simulink model "Neur_PID_sys"  (R2021a)
settings: Solver=FixedStepAuto  StartTime=0.0  StopTime=300  FixedStep=0.01  RelTol=1e-3
settings Model: Creator=WU  LastModifiedBy=WU

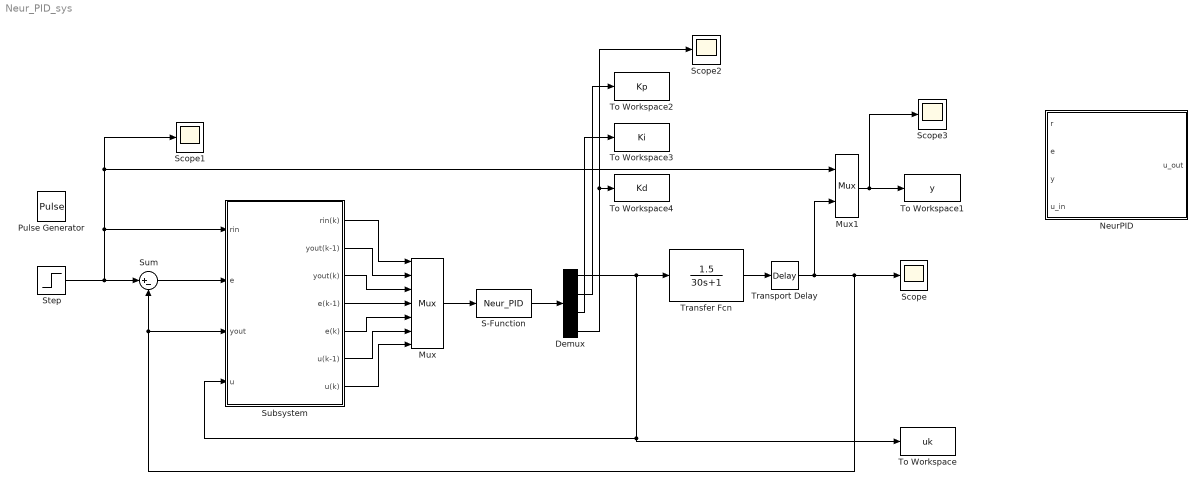
== system Neur_PID_sys ==
  Demux : Demux
  Mux : Mux  Inputs=7
  Mux1 : Mux  Inputs=2
  NeurPID : Subsystem
  Pulse Generator : DiscretePulseGenerator  PulseType=Time based  Period=10  PulseWidth=5
  S-Function : S-Function  FunctionName=Neur_PID  SFunctionDeploymentMode=off  EnableBusSupport=off
  Scope{,1..3} (4 alike) : Scope
  Step : Step  SampleTime=0  ZeroCross=off
  Subsystem : Subsystem
  Sum : Sum  Inputs=|+-
  To Workspace : ToWorkspace  VariableName=uk  SaveFormat=Structure With Time  SampleTime=-1
  To Workspace1 : ToWorkspace  VariableName=y  SaveFormat=Structure With Time  SampleTime=-1
  To Workspace2 : ToWorkspace  VariableName=Kp  SaveFormat=Structure With Time  SampleTime=-1
  To Workspace3 : ToWorkspace  VariableName=Ki  SaveFormat=Structure With Time  SampleTime=-1
  To Workspace4 : ToWorkspace  VariableName=Kd  SaveFormat=Structure With Time  SampleTime=-1
  Transfer Fcn : TransferFcn  Numerator=[1.5]  Denominator=[30 1]
  Transport Delay : TransportDelay  DelayTime=10  BufferSize=100000
  wires:
  Demux/2 -> To Workspace2/1
  Subsystem/6(u(k-1)) -> Mux/6
  Demux/3 -> To Workspace3/1
  Step/1 -> Scope1/1, Mux1/1, Subsystem/1(rin), Sum/1
  Transfer Fcn/1 -> Transport Delay/1
  Mux1/1 -> Scope3/1, To Workspace1/1
  Sum/1 -> Subsystem/2(e)
  Transport Delay/1 -> Mux1/2, Scope/1, Subsystem/3(yout), Sum/2
  Subsystem/1(rin(k)) -> Mux/1
  Subsystem/3(yout(k)) -> Mux/3
  Subsystem/5(e(k)) -> Mux/5
  Subsystem/4(e(k-1)) -> Mux/4
  Demux/1 -> Subsystem/4(u), To Workspace/1, Transfer Fcn/1
  S-Function/1 -> Demux/1
  Demux/4 -> Scope2/1, To Workspace4/1
  Subsystem/2(yout(k-1)) -> Mux/2
  Mux/1 -> S-Function/1
  Subsystem/7(u(k)) -> Mux/7

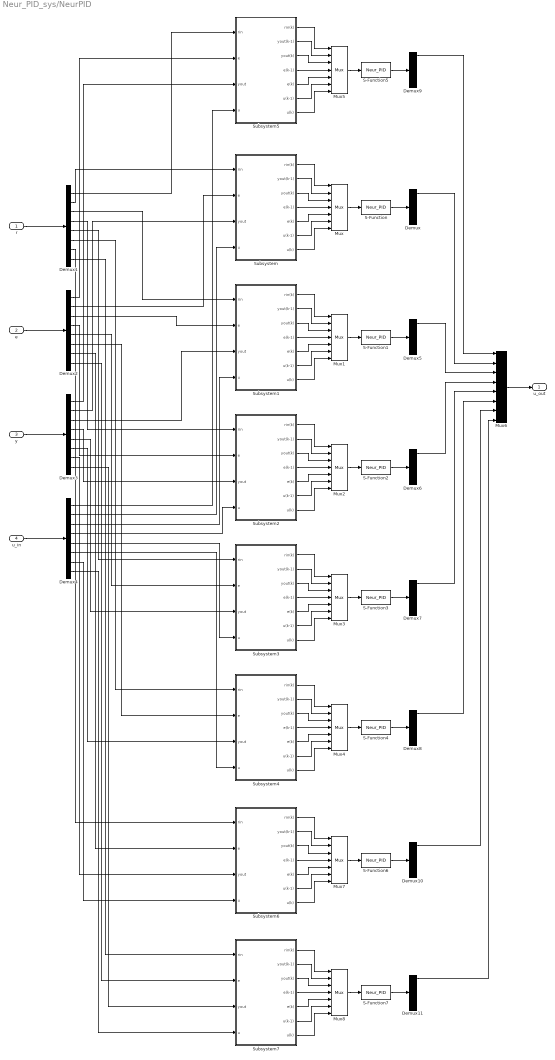
== system Neur_PID_sys/NeurPID ==
  r : Inport
  e : Inport  Port=2
  y : Inport  Port=3
  u_in : Inport  Port=4
  Demux{,5..11} (8 alike) : Demux
      settings: DisplayOption=none
  Demux{1..4} (4 alike) : Demux  Outputs=8
      settings: DisplayOption=none
  Mux{,1..5,7..8} (8 alike) : Mux  Inputs=7
  Mux6 : Mux  Inputs=8
  S-Function{,1..7} (8 alike) : S-Function  FunctionName=Neur_PID  SFunctionDeploymentMode=off  EnableBusSupport=off
  Subsystem : Subsystem
  Subsystem1 : Subsystem
  Subsystem2 : Subsystem
  Subsystem3 : Subsystem
  Subsystem4 : Subsystem
  Subsystem5 : Subsystem
  Subsystem6 : Subsystem
  Subsystem7 : Subsystem
  u_out : Outport
  wires:
  Mux/1 -> S-Function/1
  Subsystem/5(e(k)) -> Mux/5
  S-Function/1 -> Demux/1
  Subsystem/7(u(k)) -> Mux/7
  Subsystem/3(yout(k)) -> Mux/3
  Subsystem/1(rin(k)) -> Mux/1
  Subsystem/6(u(k-1)) -> Mux/6
  Subsystem/4(e(k-1)) -> Mux/4
  Subsystem/2(yout(k-1)) -> Mux/2
  r/1 -> Demux1/1
  e/1 -> Demux2/1
  y/1 -> Demux3/1
  u_in/1 -> Demux4/1
  Subsystem1/4(e(k-1)) -> Mux1/4
  Subsystem1/6(u(k-1)) -> Mux1/6
  Subsystem1/3(yout(k)) -> Mux1/3
  S-Function1/1 -> Demux5/1
  Mux1/1 -> S-Function1/1
  Subsystem1/1(rin(k)) -> Mux1/1
  Subsystem1/7(u(k)) -> Mux1/7
  Subsystem1/5(e(k)) -> Mux1/5
  Subsystem1/2(yout(k-1)) -> Mux1/2
  Subsystem2/4(e(k-1)) -> Mux2/4
  Subsystem2/6(u(k-1)) -> Mux2/6
  Subsystem2/3(yout(k)) -> Mux2/3
  S-Function2/1 -> Demux6/1
  Mux2/1 -> S-Function2/1
  Subsystem2/1(rin(k)) -> Mux2/1
  Subsystem2/7(u(k)) -> Mux2/7
  Subsystem2/5(e(k)) -> Mux2/5
  Subsystem2/2(yout(k-1)) -> Mux2/2
  Subsystem3/4(e(k-1)) -> Mux3/4
  Subsystem3/6(u(k-1)) -> Mux3/6
  Subsystem3/3(yout(k)) -> Mux3/3
  S-Function3/1 -> Demux7/1
  Mux3/1 -> S-Function3/1
  Subsystem3/1(rin(k)) -> Mux3/1
  Subsystem3/7(u(k)) -> Mux3/7
  Subsystem3/5(e(k)) -> Mux3/5
  Subsystem3/2(yout(k-1)) -> Mux3/2
  Subsystem4/4(e(k-1)) -> Mux4/4
  Subsystem4/6(u(k-1)) -> Mux4/6
  Subsystem4/3(yout(k)) -> Mux4/3
  S-Function4/1 -> Demux8/1
  Mux4/1 -> S-Function4/1
  Subsystem4/1(rin(k)) -> Mux4/1
  Subsystem4/7(u(k)) -> Mux4/7
  Subsystem4/5(e(k)) -> Mux4/5
  Subsystem4/2(yout(k-1)) -> Mux4/2
  Subsystem5/4(e(k-1)) -> Mux5/4
  Subsystem5/6(u(k-1)) -> Mux5/6
  Subsystem5/3(yout(k)) -> Mux5/3
  S-Function5/1 -> Demux9/1
  Mux5/1 -> S-Function5/1
  Subsystem5/1(rin(k)) -> Mux5/1
  Subsystem5/7(u(k)) -> Mux5/7
  Subsystem5/5(e(k)) -> Mux5/5
  Subsystem5/2(yout(k-1)) -> Mux5/2
  Demux1/1 -> Subsystem5/1(rin)
  Demux1/2 -> Subsystem/1(rin)
  Demux1/3 -> Subsystem1/1(rin)
  Demux1/4 -> Subsystem2/1(rin)
  Demux1/5 -> Subsystem3/1(rin)
  Demux1/6 -> Subsystem4/1(rin)
  Demux2/1 -> Subsystem5/2(e)
  Demux2/2 -> Subsystem/2(e)
  Demux2/3 -> Subsystem1/2(e)
  Demux2/4 -> Subsystem2/2(e)
  Demux2/5 -> Subsystem3/2(e)
  Demux2/6 -> Subsystem4/2(e)
  Demux3/1 -> Subsystem5/3(yout)
  Demux3/2 -> Subsystem/3(yout)
  Demux3/3 -> Subsystem1/3(yout)
  Demux3/4 -> Subsystem2/3(yout)
  Demux3/5 -> Subsystem3/3(yout)
  Demux3/6 -> Subsystem4/3(yout)
  Demux4/1 -> Subsystem5/4(u)
  Demux4/2 -> Subsystem/4(u)
  Demux4/3 -> Subsystem1/4(u)
  Demux4/4 -> Subsystem2/4(u)
  Demux4/5 -> Subsystem3/4(u)
  Demux4/6 -> Subsystem4/4(u)
  Mux6/1 -> u_out/1
  Demux9/1 -> Mux6/1
  Demux/1 -> Mux6/2
  Demux5/1 -> Mux6/3
  Demux6/1 -> Mux6/4
  Demux7/1 -> Mux6/5
  Demux8/1 -> Mux6/6
  Mux7/1 -> S-Function6/1
  Subsystem6/5(e(k)) -> Mux7/5
  Subsystem6/6(u(k-1)) -> Mux7/6
  Subsystem6/2(yout(k-1)) -> Mux7/2
  Subsystem6/3(yout(k)) -> Mux7/3
  Subsystem6/7(u(k)) -> Mux7/7
  Subsystem6/4(e(k-1)) -> Mux7/4
  S-Function6/1 -> Demux10/1
  Subsystem6/1(rin(k)) -> Mux7/1
  Mux8/1 -> S-Function7/1
  Subsystem7/5(e(k)) -> Mux8/5
  Subsystem7/6(u(k-1)) -> Mux8/6
  Subsystem7/2(yout(k-1)) -> Mux8/2
  Subsystem7/3(yout(k)) -> Mux8/3
  Subsystem7/7(u(k)) -> Mux8/7
  Subsystem7/4(e(k-1)) -> Mux8/4
  S-Function7/1 -> Demux11/1
  Subsystem7/1(rin(k)) -> Mux8/1
  Demux1/7 -> Subsystem6/1(rin)
  Demux2/7 -> Subsystem6/2(e)
  Demux3/7 -> Subsystem6/3(yout)
  Demux4/7 -> Subsystem6/4(u)
  Demux1/8 -> Subsystem7/1(rin)
  Demux2/8 -> Subsystem7/2(e)
  Demux3/8 -> Subsystem7/3(yout)
  Demux4/8 -> Subsystem7/4(u)
  Demux10/1 -> Mux6/7
  Demux11/1 -> Mux6/8

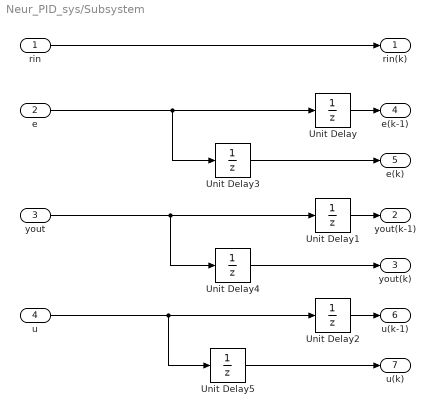
== system Neur_PID_sys/Subsystem ==
  rin : Inport
  e : Inport  Port=2
  yout : Inport  Port=3
  u : Inport  Port=4
  Unit Delay{,1..5} (6 alike) : UnitDelay  SampleTime=-1  HasFrameUpgradeWarning=on
  rin(k) : Outport
  yout(k-1) : Outport  Port=2
  yout(k) : Outport  Port=3
  e(k-1) : Outport  Port=4
  e(k) : Outport  Port=5
  u(k-1) : Outport  Port=6
  u(k) : Outport  Port=7
  wires:
  rin/1 -> rin(k)/1
  Unit Delay/1 -> e(k-1)/1
  Unit Delay1/1 -> yout(k-1)/1
  Unit Delay2/1 -> u(k-1)/1
  Unit Delay3/1 -> e(k)/1
  Unit Delay4/1 -> yout(k)/1
  Unit Delay5/1 -> u(k)/1
  e/1 -> Unit Delay/1, Unit Delay3/1
  yout/1 -> Unit Delay1/1, Unit Delay4/1
  u/1 -> Unit Delay2/1, Unit Delay5/1

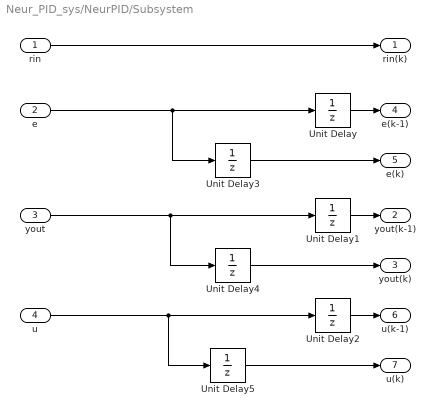
== system Neur_PID_sys/NeurPID/Subsystem ==
  rin : Inport
  e : Inport  Port=2
  yout : Inport  Port=3
  u : Inport  Port=4
  Unit Delay{,1..5} (6 alike) : UnitDelay  SampleTime=-1  HasFrameUpgradeWarning=on
  rin(k) : Outport
  yout(k-1) : Outport  Port=2
  yout(k) : Outport  Port=3
  e(k-1) : Outport  Port=4
  e(k) : Outport  Port=5
  u(k-1) : Outport  Port=6
  u(k) : Outport  Port=7
  wires:
  rin/1 -> rin(k)/1
  Unit Delay/1 -> e(k-1)/1
  Unit Delay1/1 -> yout(k-1)/1
  Unit Delay2/1 -> u(k-1)/1
  Unit Delay3/1 -> e(k)/1
  Unit Delay4/1 -> yout(k)/1
  Unit Delay5/1 -> u(k)/1
  e/1 -> Unit Delay/1, Unit Delay3/1
  yout/1 -> Unit Delay1/1, Unit Delay4/1
  u/1 -> Unit Delay2/1, Unit Delay5/1

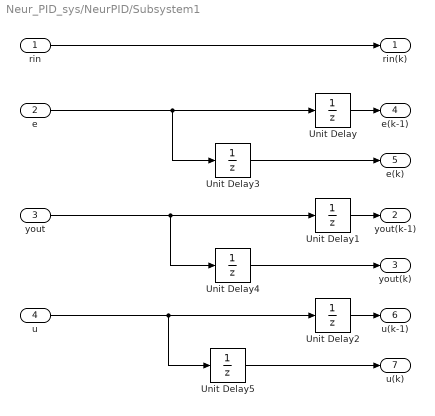
== system Neur_PID_sys/NeurPID/Subsystem1 ==
  rin : Inport
  e : Inport  Port=2
  yout : Inport  Port=3
  u : Inport  Port=4
  Unit Delay{,1..5} (6 alike) : UnitDelay  SampleTime=-1  HasFrameUpgradeWarning=on
  rin(k) : Outport
  yout(k-1) : Outport  Port=2
  yout(k) : Outport  Port=3
  e(k-1) : Outport  Port=4
  e(k) : Outport  Port=5
  u(k-1) : Outport  Port=6
  u(k) : Outport  Port=7
  wires:
  rin/1 -> rin(k)/1
  Unit Delay/1 -> e(k-1)/1
  Unit Delay1/1 -> yout(k-1)/1
  Unit Delay2/1 -> u(k-1)/1
  Unit Delay3/1 -> e(k)/1
  Unit Delay4/1 -> yout(k)/1
  Unit Delay5/1 -> u(k)/1
  e/1 -> Unit Delay/1, Unit Delay3/1
  yout/1 -> Unit Delay1/1, Unit Delay4/1
  u/1 -> Unit Delay2/1, Unit Delay5/1

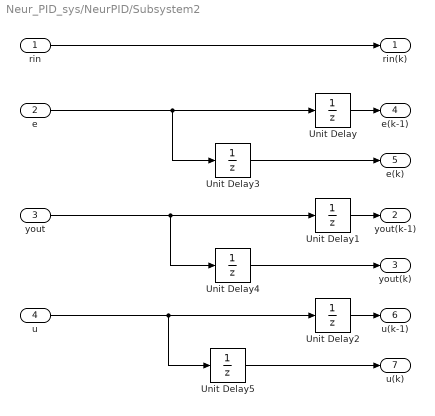
== system Neur_PID_sys/NeurPID/Subsystem2 ==
  rin : Inport
  e : Inport  Port=2
  yout : Inport  Port=3
  u : Inport  Port=4
  Unit Delay{,1..5} (6 alike) : UnitDelay  SampleTime=-1  HasFrameUpgradeWarning=on
  rin(k) : Outport
  yout(k-1) : Outport  Port=2
  yout(k) : Outport  Port=3
  e(k-1) : Outport  Port=4
  e(k) : Outport  Port=5
  u(k-1) : Outport  Port=6
  u(k) : Outport  Port=7
  wires:
  rin/1 -> rin(k)/1
  Unit Delay/1 -> e(k-1)/1
  Unit Delay1/1 -> yout(k-1)/1
  Unit Delay2/1 -> u(k-1)/1
  Unit Delay3/1 -> e(k)/1
  Unit Delay4/1 -> yout(k)/1
  Unit Delay5/1 -> u(k)/1
  e/1 -> Unit Delay/1, Unit Delay3/1
  yout/1 -> Unit Delay1/1, Unit Delay4/1
  u/1 -> Unit Delay2/1, Unit Delay5/1

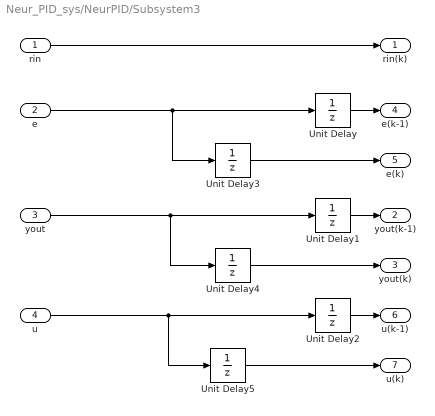
== system Neur_PID_sys/NeurPID/Subsystem3 ==
  rin : Inport
  e : Inport  Port=2
  yout : Inport  Port=3
  u : Inport  Port=4
  Unit Delay{,1..5} (6 alike) : UnitDelay  SampleTime=-1  HasFrameUpgradeWarning=on
  rin(k) : Outport
  yout(k-1) : Outport  Port=2
  yout(k) : Outport  Port=3
  e(k-1) : Outport  Port=4
  e(k) : Outport  Port=5
  u(k-1) : Outport  Port=6
  u(k) : Outport  Port=7
  wires:
  rin/1 -> rin(k)/1
  Unit Delay/1 -> e(k-1)/1
  Unit Delay1/1 -> yout(k-1)/1
  Unit Delay2/1 -> u(k-1)/1
  Unit Delay3/1 -> e(k)/1
  Unit Delay4/1 -> yout(k)/1
  Unit Delay5/1 -> u(k)/1
  e/1 -> Unit Delay/1, Unit Delay3/1
  yout/1 -> Unit Delay1/1, Unit Delay4/1
  u/1 -> Unit Delay2/1, Unit Delay5/1

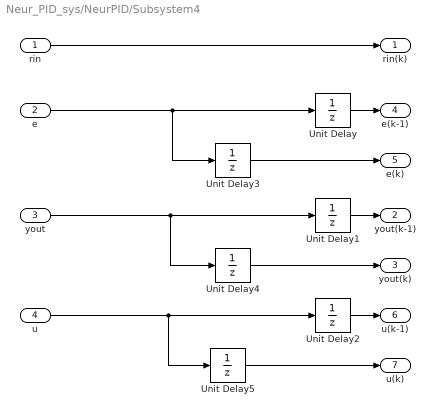
== system Neur_PID_sys/NeurPID/Subsystem4 ==
  rin : Inport
  e : Inport  Port=2
  yout : Inport  Port=3
  u : Inport  Port=4
  Unit Delay{,1..5} (6 alike) : UnitDelay  SampleTime=-1  HasFrameUpgradeWarning=on
  rin(k) : Outport
  yout(k-1) : Outport  Port=2
  yout(k) : Outport  Port=3
  e(k-1) : Outport  Port=4
  e(k) : Outport  Port=5
  u(k-1) : Outport  Port=6
  u(k) : Outport  Port=7
  wires:
  rin/1 -> rin(k)/1
  Unit Delay/1 -> e(k-1)/1
  Unit Delay1/1 -> yout(k-1)/1
  Unit Delay2/1 -> u(k-1)/1
  Unit Delay3/1 -> e(k)/1
  Unit Delay4/1 -> yout(k)/1
  Unit Delay5/1 -> u(k)/1
  e/1 -> Unit Delay/1, Unit Delay3/1
  yout/1 -> Unit Delay1/1, Unit Delay4/1
  u/1 -> Unit Delay2/1, Unit Delay5/1

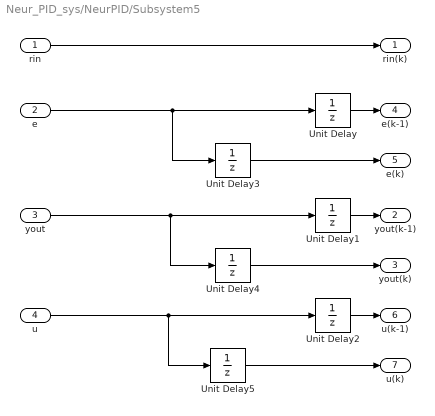
== system Neur_PID_sys/NeurPID/Subsystem5 ==
  rin : Inport
  e : Inport  Port=2
  yout : Inport  Port=3
  u : Inport  Port=4
  Unit Delay{,1..5} (6 alike) : UnitDelay  SampleTime=-1  HasFrameUpgradeWarning=on
  rin(k) : Outport
  yout(k-1) : Outport  Port=2
  yout(k) : Outport  Port=3
  e(k-1) : Outport  Port=4
  e(k) : Outport  Port=5
  u(k-1) : Outport  Port=6
  u(k) : Outport  Port=7
  wires:
  rin/1 -> rin(k)/1
  Unit Delay/1 -> e(k-1)/1
  Unit Delay1/1 -> yout(k-1)/1
  Unit Delay2/1 -> u(k-1)/1
  Unit Delay3/1 -> e(k)/1
  Unit Delay4/1 -> yout(k)/1
  Unit Delay5/1 -> u(k)/1
  e/1 -> Unit Delay/1, Unit Delay3/1
  yout/1 -> Unit Delay1/1, Unit Delay4/1
  u/1 -> Unit Delay2/1, Unit Delay5/1

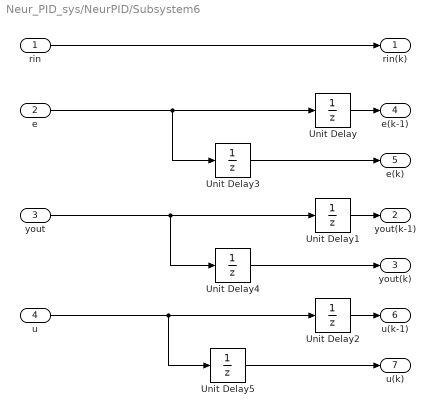
== system Neur_PID_sys/NeurPID/Subsystem6 ==
  rin : Inport
  e : Inport  Port=2
  yout : Inport  Port=3
  u : Inport  Port=4
  Unit Delay{,1..5} (6 alike) : UnitDelay  SampleTime=-1  HasFrameUpgradeWarning=on
  rin(k) : Outport
  yout(k-1) : Outport  Port=2
  yout(k) : Outport  Port=3
  e(k-1) : Outport  Port=4
  e(k) : Outport  Port=5
  u(k-1) : Outport  Port=6
  u(k) : Outport  Port=7
  wires:
  rin/1 -> rin(k)/1
  Unit Delay/1 -> e(k-1)/1
  Unit Delay1/1 -> yout(k-1)/1
  Unit Delay2/1 -> u(k-1)/1
  Unit Delay3/1 -> e(k)/1
  Unit Delay4/1 -> yout(k)/1
  Unit Delay5/1 -> u(k)/1
  e/1 -> Unit Delay/1, Unit Delay3/1
  yout/1 -> Unit Delay1/1, Unit Delay4/1
  u/1 -> Unit Delay2/1, Unit Delay5/1

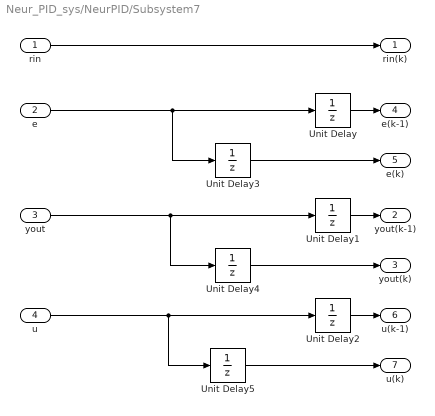
== system Neur_PID_sys/NeurPID/Subsystem7 ==
  rin : Inport
  e : Inport  Port=2
  yout : Inport  Port=3
  u : Inport  Port=4
  Unit Delay{,1..5} (6 alike) : UnitDelay  SampleTime=-1  HasFrameUpgradeWarning=on
  rin(k) : Outport
  yout(k-1) : Outport  Port=2
  yout(k) : Outport  Port=3
  e(k-1) : Outport  Port=4
  e(k) : Outport  Port=5
  u(k-1) : Outport  Port=6
  u(k) : Outport  Port=7
  wires:
  rin/1 -> rin(k)/1
  Unit Delay/1 -> e(k-1)/1
  Unit Delay1/1 -> yout(k-1)/1
  Unit Delay2/1 -> u(k-1)/1
  Unit Delay3/1 -> e(k)/1
  Unit Delay4/1 -> yout(k)/1
  Unit Delay5/1 -> u(k)/1
  e/1 -> Unit Delay/1, Unit Delay3/1
  yout/1 -> Unit Delay1/1, Unit Delay4/1
  u/1 -> Unit Delay2/1, Unit Delay5/1
